simulink model "CarteSon"  (Simulink 6.6)
settings: Solver=ode3  StartTime=0.0  StopTime=inf  RelTol=1e-3
undefined symbols (not defined in the file or in its folder): dfilt
libraries: dspwin32 x4, dspbuff3 x2, dsparch4 x1
settings Model: Creator=gbinet  LastModifiedBy=userportmfr
settings DebuggingCC: SignalResolutionControl=TryResolveAllWithWarning

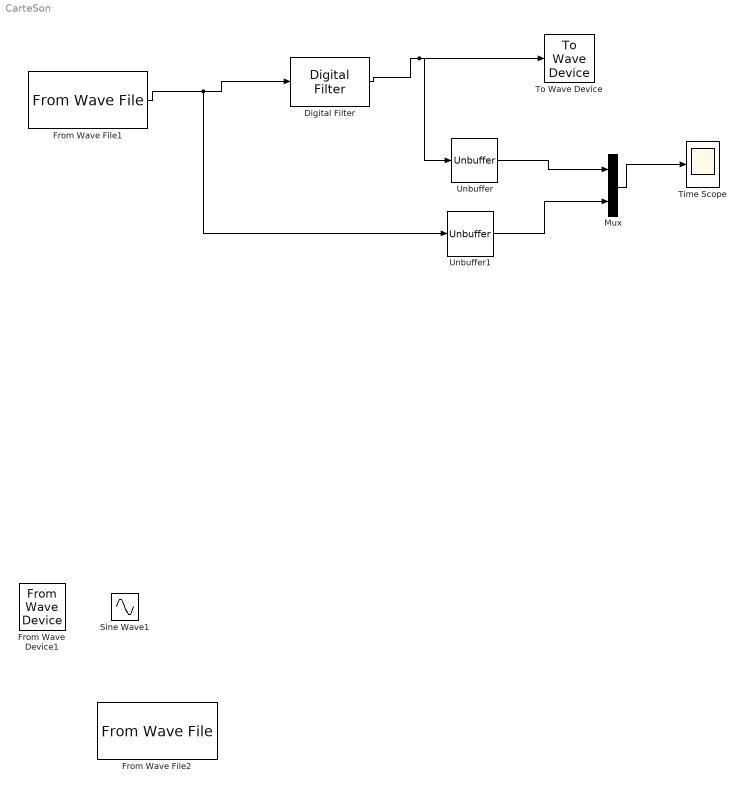
== system CarteSon ==
  Digital Filter : dsparch4/Digital Filter  DialogController=dspdialog.DigitalFilter  DialogControllerArgs=DataTag0  TypePopup=IIR (poles & zeros)  IIRFiltStruct=Direct form I  AllPoleFiltStruct=Direct form  FIRFiltStruct=Direct form  CoeffSource=Specify via dialog  NumCoeffs=NumD  DenCoeffs=DenD  BiQuadCoeffs=[1 0.3 0.4 1 0.1 0.2]  LatticeCoeffs=[0.2 0.4]  denIgnore=on  FiltPerSampPopup=One filter per frame  IC=0  ICnum=0  ICden=0  roundingMode=Floor  overflowMode=on  ScaleValues=1  scaleValueFracLength=14  stageInFracLength=15  stageOutFracLength=15  FilterSource=Specify via dialog  dfiltObjectName=dfilt.dffir([1 2 1])
  From Wave Device1 : dspwin32/From Wave Device  SampleRate=User-defined  UserRate=Fs  SampleWidth=16  Stereo=off  SamplesPerFrame=64  QueueDuration=0.1  useDefaultDevice=on  userDeviceID=SoundMAX HD Audio  dType=double
  From Wave File1 : dspwin32/From Wave File  FileName=Rokia03.wav  SamplesPerFrame=256  MinBufSize=256  dType=double  bLoop=off  timesToPlay=1  restartMode=immediately after last sample  firstSampleOutput=off  lastSampleOutput=off
  From Wave File2 : dspwin32/From Wave File  FileName=Sinus600.wav  SamplesPerFrame=256  MinBufSize=256  dType=double  bLoop=off  timesToPlay=1  restartMode=immediately after last sample  firstSampleOutput=off  lastSampleOutput=off
  Mux : Mux  Inputs=2
  Sine Wave1 : Sin  SineType=Sample based  Samples=83  SampleTime=1/8000
  Time Scope : Scope
      settings: TimeRange=0.02  YMin=-0.25  YMax=0.4  DataFormat=Structure  MaxDataPoints=50000
  To Wave Device : dspwin32/To Wave Device  bufDuration=2  determineBufSize=on  userIntBufSize=256  initDelay=0.1  useDefaultDevice=on  userDeviceID=SoundMAX HD Audio  enable24Bit=off
  Unbuffer : dspbuff3/Unbuffer  ic=0
  Unbuffer1 : dspbuff3/Unbuffer  ic=0
  wires:
  Digital Filter/1 -> Unbuffer/1, To Wave Device/1
  From Wave File1/1 -> Digital Filter/1, Unbuffer1/1
  Unbuffer/1 -> Mux/1
  Unbuffer1/1 -> Mux/2
  Mux/1 -> Time Scope/1
